simulink model "L1AdaptiveFuntionTest"  (R2015b)
settings: Solver=ode23t  SolverMode=SingleTasking  StartTime=0.0  StopTime=10  MaxStep=1e-5
InitFcn:
  | global R;
  | R = 2.875;
  | global L;
  | L = 0.00153;
  | SampleT = 1e-4;
  | R0 = 1.5;
  | L0 = 2e-3;
  | Beta1 = 10000;
  | Beta2 = 50000;
libraries: powerlib x1
Description:
  | Copyright 2008-2015 The MathWorks, Inc.
settings Model: ExtModeTrigMode=oneshot  ExtModeArmWhenConnect=off  ExtModeAutoUpdateStatusClock=off  Creator=MathWorks  LastModifiedBy=jxlllx
settings SolverCC: ZeroCrossAlgorithm=Adaptive  SolverResetMethod=Robust
settings DataIOCC: ExternalInput=[]  LimitDataPoints=off  SaveFormat=Array  SignalLoggingSaveFormat=ModelDataLogs  SaveOutput=off  SaveTime=off  SignalLoggingName=sigsOut
settings OptimizationCC: BlockReduction=off  BooleanDataType=off  ExpressionDepthLimit=2147483647  InitFltsAndDblsToZero=on  EfficientMapNaN2IntZero=off
settings DebuggingCC: UnderspecifiedInitializationDetection=Classic  MergeDetectMultiDrivingBlocksExec=none  CheckExecutionContextPreStartOutputMsg=on  CheckExecutionContextRuntimeOutputMsg=on  SignalResolutionControl=TryResolveAllWithWarning  MultiTaskDSMMsg=warning  MultiTaskCondExecSysMsg=none  SigSpecEnsureSampleTimeMsg=none  FcnCallInpInsideContextMsg=UseLocalSettings  StateNameClashWarn=warning
settings HardwareCC: ProdBitPerPointer=32  ProdLargestAtomicFloat=None  ProdIntDivRoundTo=Undefined  ProdEndianess=Unspecified  ProdWordSize=32  ProdHWDeviceType=32-bit Generic  TargetBitPerPointer=64  TargetLongLongMode=on  TargetIntDivRoundTo=Zero  TargetEndianess=LittleEndian  TargetWordSize=64  TargetHWDeviceType=MATLAB Host  ProdEqTarget=off
settings RTWCC: TargetLang=C++
settings GRTTargetCC: GeneratePreprocessorConditionals=Disable all  MultiInstanceERTCode=on  CodeInterfacePackaging=C++ class
settings ConfigComp: CovModelRefEnable=Off  CovSFcnEnable=off

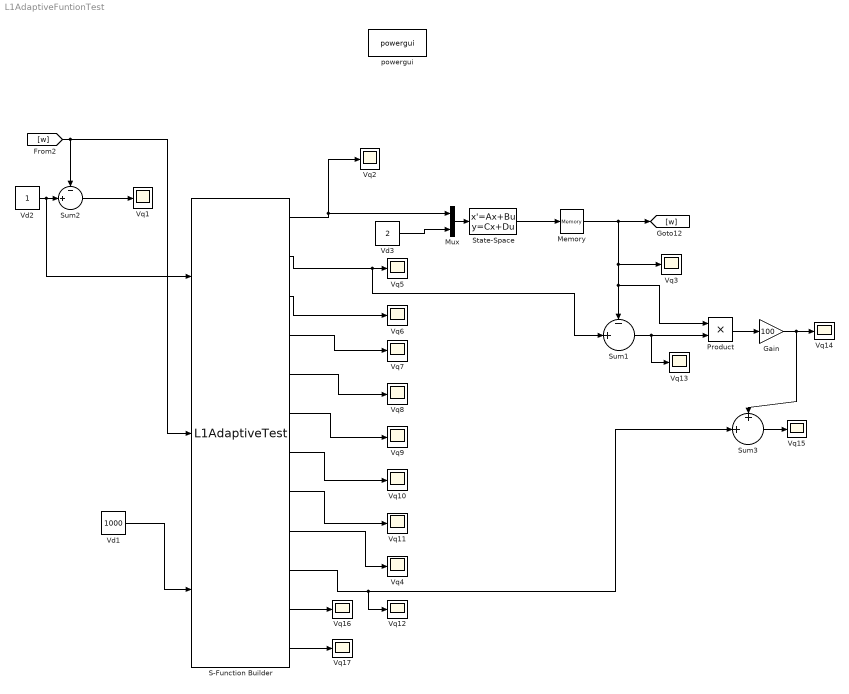
== system L1AdaptiveFuntionTest ==
  Gain : Gain  Gain=100
  Memory : Memory
  Mux : Mux  Inputs=2
  Product : Product
  S-Function Builder : S-Function  InitFcn=try, set_param(gcb,'FunctionName','L1AdaptiveTest'), end  FunctionName=L1AdaptiveTest  Parameters=0  SFunctionModules=L1AdaptiveTest_wrapper PID RL_Brain L1Adaptive  SFunctionDeploymentMode=off  EnableBusSupport=off  mask(S-Function Builder){}
      mask help: Simulink:masks:SFunctionBuilder_MD
      mask init:
      | val = [[.9  0.75 0.75 1 1 .9 .9 1]',[1 1 0.75 0.75 .9 .9 1 .9]'];try , sys = get_param(gcb,'SfunBuilderFcnName');if isempty(sys), sys = get_param(gcb,'FunctionName'); end,catch, sys = get_param(gcb,'FunctionName'); end
      settings: CopyFcn=set_param(gcbh,'LinkStatus','none')  PreSaveFcn=try, set_param(gcb,'FunctionName','L1AdaptiveTest'), end  OpenFcn=sfunctionwizard(gcbh)
      mask Display: plot(val(:,1),val(:,2)),disp(sys), port_label('input',1,'u0'), port_label('input',2,'u1'), port_label('input',3,'u2'), port_label('output',1,'Iref'), port_label('output',2,'Xest'), port_label('output',3,'Uad'), port_label('output',4,'Um'), port_label('output',5,'RefErr'), port_label('output',6,'ThetaEst'), port_label('output',7,'StateErr'), port_label('output',8,'X'), port_label('output',9,'Uref'), port_label('output',10,'AdaItem'), port_label('output',11,'West'), port_label('output',12,'SigmaEst')
  State-Space : StateSpace  A=-3  B=[1,1]  D=[0,0]  X0=0
  Sum1 : Sum  Inputs=-|+||
  Sum2 : Sum  Inputs=-|+||
  Sum3 : Sum  Inputs=+|+||
  Vd1 : Constant  Value=1000
  Vd2 : Constant
  Vd3 : Constant  Value=2
  Vq{1..17} (17 alike) : Scope
  powergui : powerlib/powergui  SimulationMode=Continuous  SolverType=Tustin  SampleTime=0  frequency=60  SPID=on  DisableSnubberDevices=off  DisableRonSwitches=off  DisableVfSwitches=off  SwTol=0  DisplayEquations=off  Interpol=off  ExternalGateDelay=off  methode=off  Ts=0  FunctionMessages=off  echomessages=off  HookPort=off  EnableUseOfTLC=off  x0status=blocks  frequencyindice=0  Pbase=100e6  ErrMax=1e-4  Iterations=50  UnitsV=kV  UnitsW=MW  buscounter=0  RestoreLinks=warning  ResistiveCurrentMeasurement=off  Frange=[0:2:500]  Ylog=off  Xlog=on  ShowGrid=off  save=off  variable=ZData  structure=0  ZoomFFT=on  StartTime=0.0  cycles=1  DisplayStyle=1  fundamental=60  FreqAxis=off  MaxFrequency=1000  frequencyindicesteady=1  RmsSteady=1  display=off
  wires:
  Vd1/1 -> S-Function Builder/3
  Vd2/1 -> S-Function Builder/1, Sum2/2
  [w] -> S-Function Builder/2, Sum2/1
  Sum2/1 -> Vq1/1
  S-Function Builder/2 -> Sum1/2, Vq5/1
  S-Function Builder/4 -> Vq7/1
  S-Function Builder/3 -> Vq6/1
  S-Function Builder/5 -> Vq8/1
  S-Function Builder/6 -> Vq9/1
  S-Function Builder/7 -> Vq10/1
  S-Function Builder/8 -> Vq11/1
  Memory/1 -> Product/1, Sum1/1, Vq3/1, [w]
  State-Space/1 -> Memory/1
  S-Function Builder/1 -> Mux/1, Vq2/1
  S-Function Builder/9 -> Vq4/1
  S-Function Builder/10 -> Sum3/2, Vq12/1
  Sum1/1 -> Product/2, Vq13/1
  Product/1 -> Gain/1
  Gain/1 -> Sum3/1, Vq14/1
  Sum3/1 -> Vq15/1
  Vd3/1 -> Mux/2
  Mux/1 -> State-Space/1
  S-Function Builder/11 -> Vq16/1
  S-Function Builder/12 -> Vq17/1
